simulink model "Power_Window0"  (R2020b)
settings: Solver=ode45  StartTime=0.0  StopTime=inf  RelTol=1e-3
PreLoadFcn:
  | OpenModel
settings Model: DataDictionary=Window_Parameter.sldd  EnablePacing=on  PacingRate=0.110000  Creator=vijay jagtap  LastModifiedBy=vijay jagtap
settings DataIOCC: SaveOutput=off  SaveTime=off

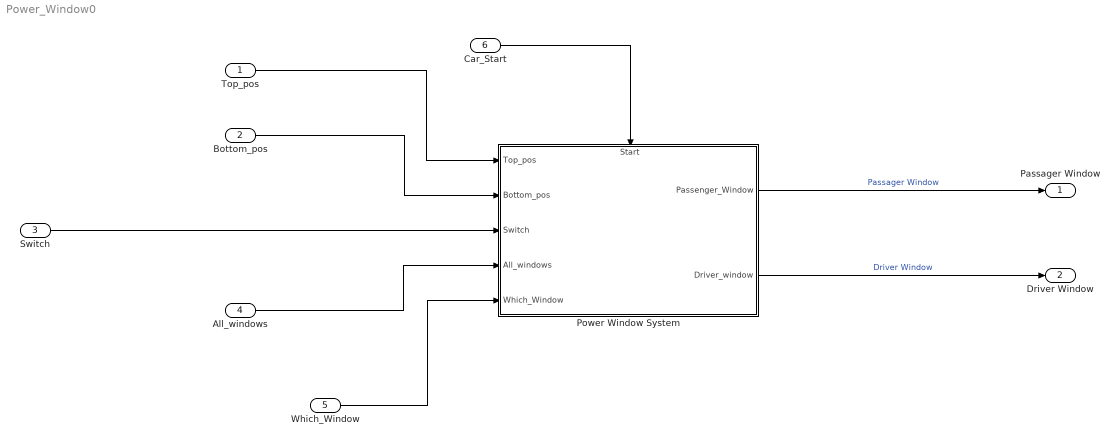
== system Power_Window0 ==
  Top_pos : Inport  OutDataTypeStr=double  PortDimensions=1
  Bottom_pos : Inport  Port=2  OutDataTypeStr=double  PortDimensions=1
  Switch : Inport  Port=3  OutDataTypeStr=double  PortDimensions=1
  All_windows : Inport  Port=4  OutDataTypeStr=double  PortDimensions=1
  Which_Window : Inport  Port=5  OutDataTypeStr=double  PortDimensions=1
  Car_Start : Inport  Port=6
  Power Window System : Stateflow chart  TreatAsAtomicUnit=on
      settings: PortSchema="{\"entries\":[{\"content\":{\"sides\":[{\"content\":{\"connectorIds\":[\"In2\",\"In3\",\"In4\",\"In5\",\"In6\"]},\"type\":\"ConnectorPlacement.EquallySpacedRectSide\",\"uuid\":\"7d301746-044d-459f-ba6b-5662a70ae466\"},{\"content\":{\"connectorIds\":[\"Out1\",\"Out2\"],\"side\":\"RIGHT\"},\"type\":\"ConnectorPlacement.EquallySpacedRectSide\",\"uuid\":\"75d7c418-4651-4950-9195-5bddf2c48ee6\"},{\"content\":{\"connectorIds\":[\"In1\"],\"side\":\"TOP\"},\"type\":\"ConnectorPlacement.EquallySpacedRectSide\",\"uuid\":\"8be66b67-2cc5-498f-a385-26e27fa49e52\"},{\"content\":{\"connectorIds\":[],\"side\":\"HIDDEN\"},\"type\":\"ConnectorPlacement.EquallySpacedRectSide\",\"uuid\":\"cb70370e-bb86-476c-bd89-087ebad211e1\"}]},\"type\":\"ConnectorPlacement.EquallySpacedConnector\",\"uuid\":\"60d77608-c50d-4f3a-9a5d-9082b7b5ccb8\"}],\"packageUris\":[\"http://schema.mathworks.com/mf0/Connector/R2020b\"],\"version\":\"1.0\"}"
  Passager Window : Outport  OutDataTypeStr=double  PortDimensions=1  SampleTime=[0,1]
  Driver Window : Outport  Port=2  OutDataTypeStr=double  PortDimensions=1  SampleTime=[0,1]
  wires:
  Switch/1 -> Power Window System/4(Switch)
  Which_Window/1 -> Power Window System/6(Which_Window)
  Top_pos/1 -> Power Window System/2(Top_pos)
  All_windows/1 -> Power Window System/5(All_windows)
  Power Window System/1(Passenger_Window) -> Passager Window/1  "Passager Window"
  Power Window System/2(Driver_window) -> Driver Window/1  "Driver Window"
  Bottom_pos/1 -> Power Window System/3(Bottom_pos)
  Car_Start/1 -> Power Window System/1(Start)

== stateflow chart Power_Window0/Power Window System ==
  state Start
  state Car_On
    state IDLE
    state DriverWindow
      (history)
      state IDLE
      state DOWN_ALL
        entry:
        yy = zz;
        during:
        if(Driver_window > Bottom_pos)
        Driver_window = Slide(xx,-1);
        xx = xx - 1;
        end
        if(Passenger_Window > Bottom_pos)
        Passenger_Window = Slide(yy,-1);
        yy = yy -1
        end
        exit:
        zz = yy;
      state UP_ALL
        entry:
        yy = zz;
        during:
        if(Driver_window < Top_pos)
        Driver_window = Slide(xx,1);
        xx = xx + 1;
        end
        if(Passenger_Window < Top_pos)
        Passenger_Window = Slide(yy,1);
        yy = yy +1;
        end
        exit:
        zz = yy;
      state UP
        during:
        if Driver_window < Top_pos
        Driver_window = Slide(xx,1);
        xx = xx + 1;
        end
      state DOWN
        during:
        if Driver_window > Bottom_pos
        Driver_window = Slide(xx,-1);
        xx = xx - 1;
        end
      (default) -> Car_On.DriverWindow.IDLE
      UP -> Car_On.DriverWindow.IDLE : [Switch == 0 || Switch == -1 || All_windows == 1]
      Car_On.DriverWindow.IDLE -> UP [order 3] : [Switch == 1 && All_windows == 0]
      DOWN -> Car_On.DriverWindow.IDLE : [Switch == 0 || Switch == 1 || All_windows == 1]
      Car_On.DriverWindow.IDLE -> DOWN [order 4] : [Switch == -1 && All_windows == 0]
      UP_ALL -> Car_On.DriverWindow.IDLE : [Switch == 0 || Switch == -1 || All_windows == 0]
      Car_On.DriverWindow.IDLE -> UP_ALL [order 1] : [Switch == 1 && All_windows == 1]
      DOWN_ALL -> Car_On.DriverWindow.IDLE : [Switch == 0 || Switch == 1 || All_windows == 0]
      Car_On.DriverWindow.IDLE -> DOWN_ALL [order 2] : [Switch == -1 && All_windows == 1]
    state Passenger1
      (history)
      state IDLE1
      state UP1
        during:
        if Passenger_Window < Top_pos
        Passenger_Window = Slide(zz,1);
        zz = zz + 1;
        end
      state DOWN1
        during:
        if Passenger_Window > Bottom_pos
        Passenger_Window = Slide(zz,-1);
        zz = zz - 1;
        end
      (default) -> IDLE1
      UP1 -> IDLE1 : [Switch == 0 || Switch == -1]
      IDLE1 -> UP1 [order 1] : [Switch == 1]
      DOWN1 -> IDLE1 : [Switch == 0 || Switch == 1]
      IDLE1 -> DOWN1 [order 2] : [Switch == -1]
    (default) -> Car_On.IDLE
    DriverWindow -> Car_On.IDLE : [Which_Window == 0]
    Car_On.IDLE -> DriverWindow [order 1] : [Which_Window == 1]
    Car_On.IDLE -> Passenger1 [order 2] : [Which_Window == 0]
    Passenger1 -> Car_On.IDLE : [Which_Window == 1]
  (default) -> Start
  Start -> Car_On : [Start == 1]
  Car_On -> Start : [Start == 0]
  data: window function_input; D_Sliding function_output; a function_input; Start input; Top_pos input; Bottom_pos input; Switch input; All_windows input; Which_Window input; Passenger_Window output =0; Driver_window output =0; xx local =0; yy local =0; zz local =0
  function D_Sliding = Slide(window,a):
    | function D_Sliding = Slide(window,a)
    | if a == -1
    |   D_Sliding = window - 1; 
    | end
    | if (a == 1)
    |   D_Sliding = window + 1;
    | end
